simulink model "B1_IEEE_13_bus"  (R2022b)
settings: Solver=ode4  StartTime=0.0  StopTime=tend  FixedStep=ts  MaxStep=0.04  RelTol=1e-3
undefined symbols (not defined in the file): C, C_601, C_602, C_603, C_604, C_605, C_606, C_607, C_bc_ESS, C_bc_PV, C_bc_SC, C_SC_set, Cf, f0, fc, fc1, ft2km, fv, Gf, Idcbase, Ilim, J, Ki_c1, Ki_v, Kp_c1, Kp_v, L_601, L_602, L_603, L_604, L_605, L_606, L_607, L_bc_ESS, L_bc_PV, L_bc_SC, L_line_ESS, L_line_PV, Lf, Pnom, Pset_ESS, Pset_inv, Pset_load, Pset_PV, Pset_SC, Qset_inv, R_601, R_602, R_603, R_604, R_605, R_606, R_607, R_bc_ESS, R_bc_PV, R_bc_SC, R_line_ESS, R_line_PV, R_line_SC, Rf ... (+23)
libraries: spsSeriesRLCBranchLib x12, spsLoadFlowBusLib x12, spsPiSectionLineLib x9, spsThreePhaseSeriesRLCLoadLib x8, spsThreePhaseVIMeasurementLib x8, spsVoltageMeasurementLib x8, cstblocks x8, spsCurrentMeasurementLib x6, spsGroundLib x6, spsMultimeterLib x6, spsPowerLib x6, spsSeriesRLCLoadLib x5
(part 1 of 2)
settings Model: Creator=The MathWorks, Inc.  LastModifiedBy=hxq19
settings SolverCC: AlgebraicLoopSolver=TrustRegion
settings DataIOCC: ExternalInput=getinputstruct(op_IEEE_13_node_5)  InitialState=getstatestruct(op_IEEE_13_node_5)  LimitDataPoints=on  SaveFormat=Array  ReturnWorkspaceOutputs=off
settings OptimizationCC: LifeSpan=inf
settings DebuggingCC: AlgebraicLoopMsg=none  FcnCallInpInsideContextMsg=warning  StateNameClashWarn=warning  SFUnexpectedBacktrackingDiag=warning  SFNoUnconditionalDefaultTransitionDiag=warning  SFExecutionAtInitializationDiag=none  SFMachineParentedDataDiag=warning
settings ModelReferenceCC: EnableRefExpFcnMdlSchedulingChecks=on  PropagateSignalLabelsOutOfModel=off
settings SFSimCC: CustomCodeUndefinedFunction=UseInterfaceOnly
settings CodeAppCC: StateflowObjectComments=on
settings SimscapeCC: SimscapeNormalizeSystem=off

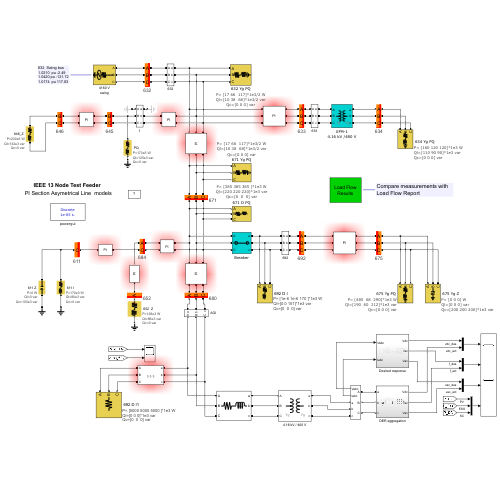
[thumbnail: Simulink's stored preview of the top-level diagram]
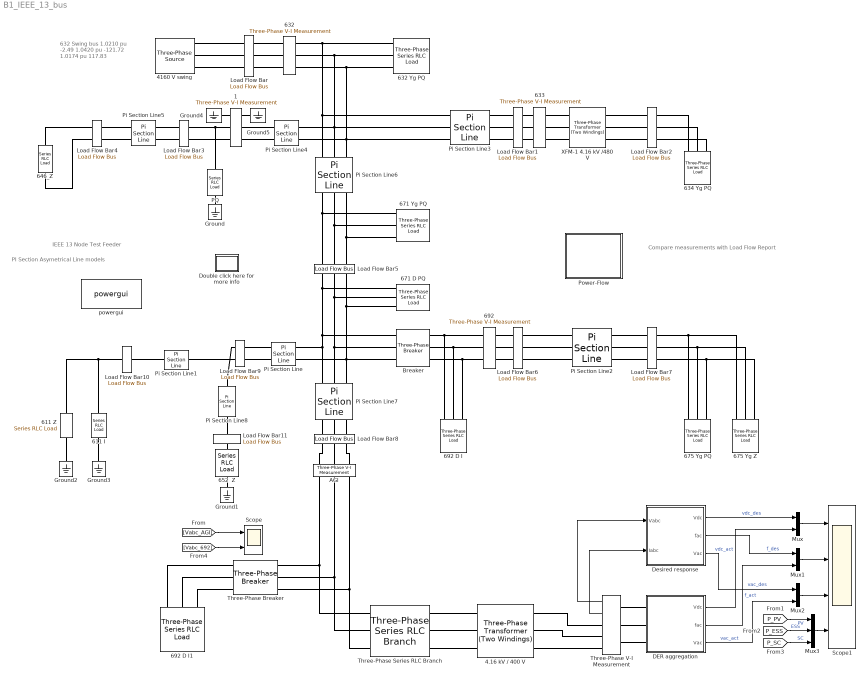
== system B1_IEEE_13_bus ==
  note: Compare measurements with
      | Load Flow Report
  note: 632 Swing bus
      | 1.0210 pu -2.49
      | 1.0420 pu -121.72
      | 1.0174 pu 117.83
  note: PI Section Asymetrical Line models
  note: IEEE 13 Node Test Feeder
  " 634 Yg PQ " : spsThreePhaseSeriesRLCLoadLib/Three-Phase Series RLC Load  LConnTagsString=A|B|C  Configuration=Y (grounded)  NominalVoltage=120e3  Vabc=[ 0.993926 1.02168 0.995885]*277.128  Vabcp=[1e3 1e3 1e3]  NominalFrequency=60  UnbalancedPower=on  ActivePower=1e+006  InductivePower=0  CapacitivePower=0  Pabc=[160 120 120]*1e3  QLabc=[110 90 90]*1e3  QCabc=[0 0 0]  Pabcp=[10e3 9e3 11e3]  QLabcp=[100 90 110]  QCabcp=[100 90 110]  Measurements=None  LoadType=constant PQ
      settings: AttributesFormatString=|
      | P= %<Pabc> W
      | Ql=%<QLabc> var
      | Qc=%<QCabc> var
  1 : spsThreePhaseVIMeasurementLib/Three-Phase V-I Measurement  VoltageMeasurement=phase-to-ground  SetLabelV=on  LabelV=Vabc_645  Vpu=off  VpuLL=off  CurrentMeasurement=yes  SetLabelI=on  LabelI=Iabc_645  Ipu=off  Pbase=100e6  Vbase=4160  OutputType=Complex  PhasorSimulation=off  PSBequivalent=0
  4.16 kV / 400 V : spsThreePhaseTransformerTwoWindingsLib/Three-Phase Transformer (Two Windings)  Winding1Connection=Yg  Winding2Connection=Yg  CoreType=Three single-phase transformers  SetSaturation=off  Hysteresis=off  DataFile='hysteresis'  SetInitialFlux=off  Measurements=None  UNITS=pu  NominalPower=[Stotal,f0]  Winding1=[ V1 , 0.001 , 0.03 ]  Winding2=[ V2 , 0.001 , 0.03 ]  Rm=500  Lm=inf  L0=0.5  Saturation=[ 0,0 ; 0.0024,1.2 ; 1.0,1.52 ]  InitialFluxes=[ 0.8 , -0.8 , 0.7 ]  BreakLoop=off  DiscreteSolver=Trapezoidal iterative  DataType=off  TransfoNumber=0
  4160 V swing : spsThreePhaseSourceLib/Three-Phase Source  InternalConnection=Yg  VoltagePhases=on  Voltage=120e3  PhaseAngle=0  Voltage_phases=[ 1.021 1.042 1.0174]*2401.78  PhaseAngles_phases=[ -2.49006 -121.72 117.83]  Frequency=60  NonIdealSource=on  SpecifyImpedance=off  Resistance=1e-5  Inductance=0  ShortCircuitLevel=100e6  BaseVoltage=120e3  XRratio=10  BusType=swing  Pref=0  Qref=0  Prefabc=[0 0 0]  Qrefabc=[0 0 0]  Qmin="[-inf  -inf -inf]"  Qmax="[inf  inf inf]"
  611 I : spsSeriesRLCLoadLib/Series RLC Load  LConnTagsString=a  RConnTagsString=__new0  NominalVoltage=0.986755*2401.78  NominalFrequency=60  ActivePower=170e3  InductivePower=80e3  CapacitivePower=0  Setx0=off  InitialVoltage=0  SetiL0=off  InitialCurrent=0  Measurements=Branch voltage and current  LoadType=constant I
      settings: AttributesFormatString=|
      | P=%<ActivePower> W
      | Ql=%<InductivePower> var
      | Qc=%<CapacitivePower> var
  611 Z : spsSeriesRLCLoadLib/Series RLC Load  LConnTagsString=a  RConnTagsString=__new0  NominalVoltage=4160/sqrt(3)  NominalFrequency=60  ActivePower=0  InductivePower=0  CapacitivePower=100e3  Setx0=off  InitialVoltage=0  SetiL0=off  InitialCurrent=0  Measurements=None  LoadType=constant Z
      settings: AttributesFormatString=|
      | P=%<ActivePower> W
      | Ql=%<InductivePower> var
      | Qc=%<CapacitivePower> var
  632 : spsThreePhaseVIMeasurementLib/Three-Phase V-I Measurement  VoltageMeasurement=phase-to-ground  SetLabelV=on  LabelV=Vabc_632  Vpu=off  VpuLL=off  CurrentMeasurement=yes  SetLabelI=on  LabelI=Iabc_632  Ipu=off  Pbase=100e6  Vbase=4160  OutputType=Complex  PhasorSimulation=off  PSBequivalent=0
  632 Yg PQ : spsThreePhaseSeriesRLCLoadLib/Three-Phase Series RLC Load  LConnTagsString=A|B|C  Configuration=Y (grounded)  NominalVoltage=120e3  Vabc=[ 1.021 1.042 1.0174]*2401.78  Vabcp=[1e3 1e3 1e3]  NominalFrequency=60  UnbalancedPower=on  ActivePower=1e+006  InductivePower=0  CapacitivePower=0  Pabc="[17 66  117]*1e3/2"  QLabc="[10 38  68]*1e3/2"  QCabc=[0 0 0]  Pabcp=[10e3 9e3 11e3]  QLabcp=[100 90 110]  QCabcp=[100 90 110]  Measurements=None  LoadType=constant PQ
      settings: AttributesFormatString=|
      | P= %<Pabc> W
      | Ql=%<QLabc> var
      | Qc=%<QCabc> var
  633 : spsThreePhaseVIMeasurementLib/Three-Phase V-I Measurement  VoltageMeasurement=phase-to-ground  SetLabelV=on  LabelV=Vabc_633  Vpu=off  VpuLL=off  CurrentMeasurement=yes  SetLabelI=on  LabelI=Iabc_633  Ipu=off  Pbase=100e6  Vbase=4160  OutputType=Complex  PhasorSimulation=off  PSBequivalent=0
  646_Z : spsSeriesRLCLoadLib/Series RLC Load  LConnTagsString=a  RConnTagsString=__new0  NominalVoltage=4160  NominalFrequency=60  ActivePower=230e3  InductivePower=132e3  CapacitivePower=0  Setx0=off  InitialVoltage=0  SetiL0=off  InitialCurrent=0  Measurements=None  LoadType=constant Z
      settings: AttributesFormatString=|
      | P=%<ActivePower> W
      | Ql=%<InductivePower> var
      | Qc=%<CapacitivePower> var
  "652  Z " : spsSeriesRLCLoadLib/Series RLC Load  LConnTagsString=a  RConnTagsString=__new0  NominalVoltage=4160/sqrt(3)  NominalFrequency=60  ActivePower=128e3  InductivePower=86e3  CapacitivePower=0  Setx0=off  InitialVoltage=0  SetiL0=off  InitialCurrent=0  Measurements=None  LoadType=constant Z
      settings: AttributesFormatString=|
      | P=%<ActivePower> W
      | Ql=%<InductivePower> var
      | Qc=%<CapacitivePower> var
  671 D PQ : spsThreePhaseSeriesRLCLoadLib/Three-Phase Series RLC Load  LConnTagsString=A|B|C  Configuration=Delta  NominalVoltage=120e3  Vabc="[1  1  1]*120e3/sqrt(3)"  Vabcp=[ 1.7426 1.77325 1.71534]*2401.78  NominalFrequency=60  UnbalancedPower=on  ActivePower=1e+006  InductivePower=0  CapacitivePower=0  Pabc="[17 66  117]*1e3/2"  QLabc="[10 38  68]*1e3/2"  QCabc=[0 0 0]  Pabcp=[385 385 385 ]*1e3  QLabcp=[220 220 220]*1e3  QCabcp="[0  0  0]"  Measurements=Branch voltages and currents  LoadType=constant PQ
      settings: AttributesFormatString=|
      | P= %<Pabcp> W
      | Ql=%<QLabcp> var
      | Qc=%<QCabcp> var
  671 Yg PQ : spsThreePhaseSeriesRLCLoadLib/Three-Phase Series RLC Load  LConnTagsString=A|B|C  Configuration=Y (grounded)  NominalVoltage=120e3  Vabc=[ 0.990007 1.05293 0.977696]*2401.78  Vabcp=[1e3 1e3 1e3]  NominalFrequency=60  UnbalancedPower=on  ActivePower=1e+006  InductivePower=0  CapacitivePower=0  Pabc="[17 66  117]*1e3/2"  QLabc="[10 38  68]*1e3/2"  QCabc=[0 0 0]  Pabcp=[10e3 9e3 11e3]  QLabcp=[100 90 110]  QCabcp=[100 90 110]  Measurements=None  LoadType=constant PQ
      settings: AttributesFormatString=|
      | P= %<Pabc> W
      | Ql=%<QLabc> var
      | Qc=%<QCabc> var
  675 Yg PQ : spsThreePhaseSeriesRLCLoadLib/Three-Phase Series RLC Load  LConnTagsString=A|B|C  Configuration=Y (grounded)  NominalVoltage=120e3  Vabc=[ 0.983621 1.05532 0.975578]*2401.78  Vabcp=[1e3 1e3 1e3]  NominalFrequency=60  UnbalancedPower=on  ActivePower=1e+006  InductivePower=0  CapacitivePower=0  Pabc="[485  68  290]*1e3"  QLabc="[190  60  212]*1e3"  QCabc=[0 0 0]  Pabcp=[10e3 9e3 11e3]  QLabcp=[100 90 110]  QCabcp=[100 90 110]  Measurements=Branch voltages and currents  LoadType=constant PQ
      settings: AttributesFormatString=|
      | P= %<Pabc> W
      | Ql=%<QLabc> var
      | Qc=%<QCabc> var
  675 Yg Z : spsThreePhaseSeriesRLCLoadLib/Three-Phase Series RLC Load  LConnTagsString=A|B|C  Configuration=Y (grounded)  NominalVoltage=120e3  Vabc="[1  1  1]*4160/sqrt(3)"  Vabcp=[1e3 1e3 1e3]  NominalFrequency=60  UnbalancedPower=on  ActivePower=1e+006  InductivePower=0  CapacitivePower=0  Pabc=[0 0 0]  QLabc=[0 0 0]  QCabc=[200 200 200]*1e3  Pabcp=[10e3 9e3 11e3]  QLabcp=[100 90 110]  QCabcp=[100 90 110]  Measurements=None  LoadType=constant Z
      settings: AttributesFormatString=|
      | P= %<Pabc> W
      | Ql=%<QLabc> var
      | Qc=%<QCabc> var
  692 : spsThreePhaseVIMeasurementLib/Three-Phase V-I Measurement  VoltageMeasurement=phase-to-ground  SetLabelV=on  LabelV=Vabc_692  Vpu=off  VpuLL=off  CurrentMeasurement=yes  SetLabelI=on  LabelI=Iabc_692  Ipu=off  Pbase=100e6  Vbase=4160  OutputType=Complex  PhasorSimulation=off  PSBequivalent=0
  692 D I : spsThreePhaseSeriesRLCLoadLib/Three-Phase Series RLC Load  LConnTagsString=A|B|C  Configuration=Delta  NominalVoltage=120e3  Vabc="[1  1  1]*120e3/sqrt(3)"  Vabcp=[ 1.73731 1.75253 1.72367]*2401.78  NominalFrequency=60  UnbalancedPower=on  ActivePower=1e+006  InductivePower=0  CapacitivePower=0  Pabc="[17 66  117]*1e3/2"  QLabc="[10 38  68]*1e3/2"  QCabc=[0 0 0]  Pabcp=[1e-6 1e-6 170 ]*1e3  QLabcp=[0 0 151]*1e3  QCabcp="[0  0  0]"  Measurements=Branch voltages and currents  LoadType=constant I
      settings: AttributesFormatString=|
      | P= %<Pabcp> W
      | Ql=%<QLabcp> var
      | Qc=%<QCabcp> var
  692 D I1 : spsThreePhaseSeriesRLCLoadLib/Three-Phase Series RLC Load  LConnTagsString=A|B|C  Configuration=Delta  NominalVoltage=120e3  Vabc="[1  1  1]*120e3/sqrt(3)"  Vabcp=[ 1.73731 1.75253 1.72367]*2401.78  NominalFrequency=60  UnbalancedPower=on  ActivePower=1e+006  InductivePower=0  CapacitivePower=0  Pabc="[17 66  117]*1e3/2"  QLabc="[10 38  68]*1e3/2"  QCabc=[0 0 0]  Pabcp=[5000 5000 5000 ]*1e3  QLabcp=[0 0 0]*1e3  QCabcp="[0  0  0]"  Measurements=Branch voltages and currents  LoadType=constant I
      settings: AttributesFormatString=|
      | P= %<Pabcp> W
      | Ql=%<QLabcp> var
      | Qc=%<QCabcp> var
  AGI : spsThreePhaseVIMeasurementLib/Three-Phase V-I Measurement  VoltageMeasurement=phase-to-ground  SetLabelV=on  LabelV=Vabc_AGI  Vpu=off  VpuLL=off  CurrentMeasurement=yes  SetLabelI=on  LabelI=Iabc_AGI  Ipu=off  Pbase=100e6  Vbase=4160  OutputType=Complex  PhasorSimulation=off  PSBequivalent=0
  Breaker : spsThreePhaseBreakerLib/Three-Phase Breaker  InitialState=closed  SwitchA=off  SwitchB=off  SwitchC=off  SwitchTimes=[0.5 ]  External=off  BreakerResistance=0.0001  SnubberResistance=inf  SnubberCapacitance=0  Measurements=None
  DER aggregation : Subsystem
      settings: PortSchema="{\"entries\":[{\"content\":{\"sides\":[{\"content\":{\"connectorIds\":[\"Out1\",\"Out2\",\"Out3\"]},\"type\":\"ConnectorPlacement.EquallySpacedRectSide\",\"uuid\":\"d17645c7-cdec-4633-b3c6-cd15445995c3\"},{\"content\":{\"connectorIds\":[\"RConn1\",\"RConn2\",\"RConn3\"],\"side\":\"RIGHT\"},\"type\":\"ConnectorPlacement.EquallySpacedRectSide\",\"uuid\":\"25a3cf30-901e-4740-a075-3c8408526c60\"},{\"content\":{\"connectorIds\":[],\"side\":\"TOP\"},\"type\":\"ConnectorPlacement.EquallySpacedRectSide\",\"uuid\":\"8cde02ff-980e-4e20-bc67-22f4d69f4d72\"}]},\"type\":\"ConnectorPlacement.EquallySpacedConnector\",\"uuid\":\"2536287c-4269-40cd-b41b-6d4dfba348bd\"}],\"packageUris\":[\"http://schema.mathworks.com/mf0/Connector/R2020b\"],\"version\":\"1.0\"}"
  Desired response : Subsystem
      settings: PortSchema="{\"entries\":[{\"content\":{\"sides\":[{\"content\":{\"connectorIds\":[\"Out1\",\"Out2\",\"Out3\"]},\"type\":\"ConnectorPlacement.EquallySpacedRectSide\",\"uuid\":\"d17645c7-cdec-4633-b3c6-cd15445995c3\"},{\"content\":{\"connectorIds\":[\"In1\",\"In2\"],\"side\":\"RIGHT\"},\"type\":\"ConnectorPlacement.EquallySpacedRectSide\",\"uuid\":\"25a3cf30-901e-4740-a075-3c8408526c60\"},{\"content\":{\"connectorIds\":[],\"side\":\"TOP\"},\"type\":\"ConnectorPlacement.EquallySpacedRectSide\",\"uuid\":\"8cde02ff-980e-4e20-bc67-22f4d69f4d72\"}]},\"type\":\"ConnectorPlacement.EquallySpacedConnector\",\"uuid\":\"2536287c-4269-40cd-b41b-6d4dfba348bd\"}],\"packageUris\":[\"http://schema.mathworks.com/mf0/Connector/R2020b\"],\"version\":\"1.0\"}"
  Double click here for more info : Subsystem
      settings: OpenFcn=showdemo(bdroot(gcb))
      mask Display: disp('?')
  Ground{,1..5} (6 alike) : spsGroundLib/Ground  LConnTagsString=a
  Load Flow Bar : spsLoadFlowBusLib/Load Flow Bus  LConnTagsString=a|b|c  RConnTagsString=a|b|c  Phases=ABC  Connectors=on both sides  ID=632  Vbase=4160/sqrt(3)  Vref="[ 1.0210  1.0420  1.0174]"  Vangle="[ -2.49  -121.72  117.83]"  VLF=1.021  VLFb=1.042  VLFc=1.017  angleLF=-2.49  angleLFb=-121.7  angleLFc=117.8
      settings: AttributesFormatString=%<ID>
  Load Flow Bar1 : spsLoadFlowBusLib/Load Flow Bus  LConnTagsString=a|b|c  RConnTagsString=a|b|c  Phases=ABC  Connectors=on both sides  ID=633  Vbase=4160/sqrt(3)  Vref=[1.0 1.0 1.0]  Vangle=[0 -120 120]  VLF=1.018  VLFb=1.04  VLFc=1.015  angleLF=-2.555  angleLFb=-121.8  angleLFc=117.8
      settings: AttributesFormatString=%<ID>
  Load Flow Bar10 : spsLoadFlowBusLib/Load Flow Bus  LConnTagsString=a  RConnTagsString=a  Phases=C  Connectors=on both sides  ID=611  Vbase=4160/sqrt(3)  Vref=1.0  Vangle=0  VLF=NaN  VLFb=NaN  VLFc=0.9737  angleLF=NaN  angleLFb=NaN  angleLFc=115.8
      settings: AttributesFormatString=%<ID>
  Load Flow Bar11 : spsLoadFlowBusLib/Load Flow Bus  LConnTagsString=a  RConnTagsString=a  Phases=A  Connectors=on both sides  ID=652  Vbase=4160/sqrt(3)  Vref=1.0  Vangle=0  VLF=0.9825  VLFb=NaN  VLFc=NaN  angleLF=-5.246  angleLFb=NaN  angleLFc=NaN
      settings: AttributesFormatString=%<ID>
  Load Flow Bar2 : spsLoadFlowBusLib/Load Flow Bus  LConnTagsString=a|b|c  RConnTagsString=a|b|c  Phases=ABC  Connectors=on both sides  ID=634  Vbase=480/sqrt(3)  Vref=[1.0 1.0 1.0]  Vangle=[0 -120 120]  VLF=0.9939  VLFb=1.022  VLFc=0.9959  angleLF=-3.232  angleLFb=-122.2  angleLFc=117.3
      settings: AttributesFormatString=%<ID>
  Load Flow Bar3 : spsLoadFlowBusLib/Load Flow Bus  LConnTagsString=a|b  RConnTagsString=a|b  Phases=BC  Connectors=on both sides  ID=645  Vbase=4160/sqrt(3)  Vref=[1.0 1.0 ]  Vangle=[0 0]  VLF=NaN  VLFb=1.033  VLFc=1.015  angleLF=NaN  angleLFb=-121.9  angleLFc=117.9
      settings: AttributesFormatString=%<ID>
  Load Flow Bar4 : spsLoadFlowBusLib/Load Flow Bus  LConnTagsString=a|b  RConnTagsString=a|b  Phases=BC  Connectors=on both sides  ID=646  Vbase=4160/sqrt(3)  Vref=[1.0 1.0 ]  Vangle=[0 0]  VLF=NaN  VLFb=1.031  VLFc=1.013  angleLF=NaN  angleLFb=-122  angleLFc=117.9
      settings: AttributesFormatString=%<ID>
  Load Flow Bar5 : spsLoadFlowBusLib/Load Flow Bus  LConnTagsString=a|b|c  RConnTagsString=a|b|c  Phases=ABC  Connectors=on both sides  ID=671  Vbase=4160/sqrt(3)  Vref=[1.0 1.0 1.0]  Vangle=[0 -120 120]  VLF=0.99  VLFb=1.053  VLFc=0.9777  angleLF=-5.298  angleLFb=-122.3  angleLFc=116
      settings: AttributesFormatString=%<ID>
  Load Flow Bar6 : spsLoadFlowBusLib/Load Flow Bus  LConnTagsString=a|b|c  RConnTagsString=a|b|c  Phases=ABC  Connectors=on both sides  ID=692  Vbase=4160/sqrt(3)  Vref=[1.0 1.0 1.0]  Vangle=[0 -120 120]  VLF=0.99  VLFb=1.053  VLFc=0.9777  angleLF=-5.298  angleLFb=-122.3  angleLFc=116
      settings: AttributesFormatString=%<ID>
  Load Flow Bar7 : spsLoadFlowBusLib/Load Flow Bus  LConnTagsString=a|b|c  RConnTagsString=a|b|c  Phases=ABC  Connectors=on both sides  ID=675  Vbase=4160/sqrt(3)  Vref=[1.0 1.0 1.0]  Vangle=[0 -120 120]  VLF=0.9836  VLFb=1.055  VLFc=0.9756  angleLF=-5.544  angleLFb=-122.5  angleLFc=116
      settings: AttributesFormatString=%<ID>
  Load Flow Bar8 : spsLoadFlowBusLib/Load Flow Bus  LConnTagsString=a|b|c  RConnTagsString=a|b|c  Phases=ABC  Connectors=on both sides  ID=680  Vbase=4160/sqrt(3)  Vref=[1.0 1.0 1.0]  Vangle=[0 -120 120]  VLF=0.99  VLFb=1.053  VLFc=0.9777  angleLF=-5.298  angleLFb=-122.3  angleLFc=116
      settings: AttributesFormatString=%<ID>
  Load Flow Bar9 : spsLoadFlowBusLib/Load Flow Bus  LConnTagsString=a|b  RConnTagsString=a|b  Phases=AC  Connectors=on both sides  ID=684  Vbase=4160/sqrt(3)  Vref=[1.0 1.0 ]  Vangle=[0 -120 ]  VLF=0.9881  VLFb=NaN  VLFc=0.9757  angleLF=-5.321  angleLFb=NaN  angleLFc=115.9
      settings: AttributesFormatString=%<ID>
  Mux : Mux  Inputs=2
  Mux1 : Mux  Inputs=2
  Mux2 : Mux  Inputs=2
  Mux3 : Mux  Inputs=3
  PQ : spsSeriesRLCLoadLib/Series RLC Load  LConnTagsString=a  RConnTagsString=__new0  NominalVoltage=1.03283*2401.78  NominalFrequency=60  ActivePower=170e3  InductivePower=125e3  CapacitivePower=0  Setx0=off  InitialVoltage=0  SetiL0=off  InitialCurrent=0  Measurements=None  LoadType=constant PQ
      settings: AttributesFormatString=|
      | P=%<ActivePower> W
      | Ql=%<InductivePower> var
      | Qc=%<CapacitivePower> var
  Pi Section Line : spsPiSectionLineLib/Pi Section Line  LConnTagsString=1|i2  RConnTagsString=1|o2  Phases=2  PiSections=1  Length=300*ft2km  Frequency=60  Resistance=R_604([1 3],[1 3])  Inductance=L_604([1 3],[1 3])  Capacitance=C_604([1 3],[1 3])  SpecifyConductance=off  Conductance=0  Measurements=None  Measurements2=None
      settings: LibrarySourceBlock=sps_lib/Power Grid Elements/Pi Section Line
  Pi Section Line1 : spsPiSectionLineLib/Pi Section Line  LConnTagsString=1  RConnTagsString=1  Phases=1  PiSections=1  Length=300*ft2km  Frequency=60  Resistance=R_605(3,3)  Inductance=L_605(3,3)  Capacitance=C_605(3,3)  SpecifyConductance=off  Conductance=0  Measurements=None  Measurements2=None
      settings: LibrarySourceBlock=sps_lib/Power Grid Elements/Pi Section Line
  Pi Section Line2 : spsPiSectionLineLib/Pi Section Line  LConnTagsString=1|i2|i3  RConnTagsString=1|o2|o3  Phases=3  PiSections=1  Length=500*ft2km  Frequency=60  Resistance=R_606  Inductance=L_606  Capacitance=C_606  SpecifyConductance=off  Conductance=0  Measurements=None  Measurements2=None
      settings: LibrarySourceBlock=sps_lib/Power Grid Elements/Pi Section Line
  Pi Section Line3 : spsPiSectionLineLib/Pi Section Line  LConnTagsString=1|i2|i3  RConnTagsString=1|o2|o3  Phases=3  PiSections=1  Length=500*ft2km  Frequency=60  Resistance=R_602  Inductance=L_602  Capacitance=C_602  SpecifyConductance=off  Conductance=0  Measurements=None  Measurements2=None
      settings: LibrarySourceBlock=sps_lib/Power Grid Elements/Pi Section Line
  Pi Section Line4 : spsPiSectionLineLib/Pi Section Line  LConnTagsString=1|i2  RConnTagsString=1|o2  Phases=2  PiSections=1  Length=500*ft2km  Frequency=60  Resistance=R_603(2:3,2:3)  Inductance=L_603(2:3,2:3)  Capacitance=C_603(2:3,2:3)  SpecifyConductance=off  Conductance=0  Measurements=None  Measurements2=None
      settings: LibrarySourceBlock=sps_lib/Power Grid Elements/Pi Section Line
  Pi Section Line5 : spsPiSectionLineLib/Pi Section Line  LConnTagsString=1|i2  RConnTagsString=1|o2  Phases=2  PiSections=1  Length=300*ft2km  Frequency=60  Resistance=R_603(2:3,2:3)  Inductance=L_603(2:3,2:3)  Capacitance=C_603(2:3,2:3)  SpecifyConductance=off  Conductance=0  Measurements=None  Measurements2=None
      settings: LibrarySourceBlock=sps_lib/Power Grid Elements/Pi Section Line
  Pi Section Line6 : spsPiSectionLineLib/Pi Section Line  LConnTagsString=1|i2|i3  RConnTagsString=1|o2|o3  Phases=3  PiSections=1  Length=2000*ft2km  Frequency=60  Resistance=R_601  Inductance=L_601  Capacitance=C_601  SpecifyConductance=off  Conductance=0  Measurements=None  Measurements2=None
      settings: LibrarySourceBlock=sps_lib/Power Grid Elements/Pi Section Line
  Pi Section Line7 : spsPiSectionLineLib/Pi Section Line  LConnTagsString=1|i2|i3  RConnTagsString=1|o2|o3  Phases=3  PiSections=1  Length=1000*ft2km  Frequency=60  Resistance=R_601  Inductance=L_601  Capacitance=C_601  SpecifyConductance=off  Conductance=0  Measurements=None  Measurements2=None
      settings: LibrarySourceBlock=sps_lib/Power Grid Elements/Pi Section Line
  Pi Section Line8 : spsPiSectionLineLib/Pi Section Line  LConnTagsString=1  RConnTagsString=1  Phases=1  PiSections=1  Length=800*ft2km  Frequency=60  Resistance=R_607(1,1)  Inductance=L_607(1,1)  Capacitance=C_607(1,1)  SpecifyConductance=off  Conductance=0  Measurements=None  Measurements2=None
      settings: LibrarySourceBlock=sps_lib/Power Grid Elements/Pi Section Line
  Power-Flow : Subsystem
      mask Display: disp('Load Flow\nResults')
  Scope : Scope  NumInputPorts=2
  Scope1 : Scope  NumInputPorts=4
  Three-Phase Series RLC Branch : spsThreePhaseSeriesRLCBranchLib/Three-Phase Series RLC Branch  LConnTagsString=A|B|C  RConnTagsString=A|B|C  BranchType=RL  Resistance=Rg*Zbase  Inductance=Zg*Zbase/w0  Capacitance=1e-6  Measurements=None
  Three-Phase V-I Measurement : spsThreePhaseVIMeasurementLib/Three-Phase V-I Measurement  VoltageMeasurement=phase-to-ground  SetLabelV=off  LabelV=Vabc  Vpu=off  VpuLL=off  CurrentMeasurement=yes  SetLabelI=off  LabelI=Iabc  Ipu=off  Pbase=Sbase  Vbase=V2  OutputType=Complex  PhasorSimulation=off  PSBequivalent=0
  Three-Phase Breaker : spsThreePhaseBreakerLib/Three-Phase Breaker  InitialState=open  SwitchA=on  SwitchB=on  SwitchC=on  SwitchTimes="[tdist  trcv]"  External=off  BreakerResistance=0.01  SnubberResistance=1e6  SnubberCapacitance=inf  Measurements=None
  XFM-1 4.16 kV /480 V : spsThreePhaseTransformerTwoWindingsLib/Three-Phase Transformer (Two Windings)  Winding1Connection=Yg  Winding2Connection=Yg  CoreType=Three single-phase transformers  SetSaturation=off  Hysteresis=off  DataFile='hysteresis'  SetInitialFlux=off  Measurements=None  UNITS=pu  NominalPower=[ 500e3 , 60 ]  Winding1=[4160 0.011 0.02]  Winding2=[480 0 0]  Rm=500  Lm=500  L0=0.5  Saturation=[0 0;0.0024 1.2;1 1.52]  InitialFluxes=[0.8 -0.8 0.7]  BreakLoop=off  DiscreteSolver=Trapezoidal iterative  DataType=off  TransfoNumber=1
  powergui : spspowerguiLib/powergui  Priority=1  SimulationMode=Discrete  SampleTime=1e-5  frequency=60  Iterations=50  frequencyindice=60  Pbase=100e3  ErrMax=0.0001  UnitsV=kV  UnitsW=kW  buscounter=0  FunctionMessages=off  echomessages=off  EnableUseOfTLC=off  CurrentSourceSwitches=off  DisableSnubberDevices=off  DisableRonSwitches=off  DisableVfSwitches=off  DisplayEquations=off  AutomaticDiscreteSolvers=off  SolverType=Tustin/Backward Euler (TBE)  Interpol=off  ExternalGateDelay=off  methode=off  Ts=0  x0status=blocks  SPID=off  SwTol=0  HookPort=off  NonlinearTolerance=1e-4  nMaxIteration=100  ContinueOnMaxIteration=off  RestoreLinks=warning  ResistiveCurrentMeasurement=off  Frange=[0:2:500]  Ylog=off  Xlog=on  ShowGrid=off  save=off  variable=ZData  structure=0  ZoomFFT=on  StartTime=0.0  cycles=1  DisplayStyle=1  fundamental=60  FreqAxis=off  MaxFrequency=1000  frequencyindicesteady=1  RmsSteady=1  display=off
  wires:
  [Vabc_AGI] -> Scope/1
  [P_SC] -> Mux3/3  "SC"
  DER aggregation/1(Vdc) -> Mux/2  "vdc_act"
  DER aggregation/2(fac) -> Mux1/2  "f_act"
  Mux3/1 -> Scope1/4
  Three-Phase V-I Measurement/1 -> Desired response/1(Vabc)
  [P_PV] -> Mux3/1  "PV"
  [P_ESS] -> Mux3/2  "ESS"
  DER aggregation/3(Vac) -> Mux2/2  "vac_act"
  Mux/1 -> Scope1/1
  Mux1/1 -> Scope1/2
  Desired response/2(fac) -> Mux1/1  "f_des"
  Desired response/3(Vac) -> Mux2/1  "vac_des"
  Desired response/1(Vdc) -> Mux/1  "vdc_des"
  Mux2/1 -> Scope1/3
  Three-Phase V-I Measurement/2 -> Desired response/2(Iabc)
  [Vabc_692] -> Scope/2
  connections:
  632/RConn2 -- 632 Yg PQ/LConn2 -- Pi Section Line4/RConn1 -- Pi Section Line6/LConn2 -- Pi Section Line3/LConn2
  675 Yg Z/LConn1 -- Load Flow Bar7/LConn1 -- 675 Yg PQ/LConn1
  671 D PQ/LConn2 -- Breaker/LConn2 -- Pi Section Line7/LConn2 -- Load Flow Bar5/RConn2
  Breaker/RConn3 -- 692 D I/LConn3 -- 692/LConn3
  Pi Section Line/RConn1 -- Pi Section Line7/LConn1 -- 671 D PQ/LConn1 -- Load Flow Bar5/RConn1 -- Breaker/LConn1
  Load Flow Bar3/RConn1 -- 1/LConn2 -- PQ/LConn1
  675 Yg Z/LConn3 -- Load Flow Bar7/LConn3 -- 675 Yg PQ/LConn3
  671 Yg PQ/LConn2 -- Load Flow Bar5/LConn2 -- Pi Section Line6/RConn2
  Load Flow Bar10/LConn1 -- 611 Z/LConn1 -- 611 I/LConn1
  671 Yg PQ/LConn3 -- Load Flow Bar5/LConn3 -- Pi Section Line6/RConn3
  Pi Section Line6/LConn1 -- 632 Yg PQ/LConn1 -- 632/RConn1 -- Pi Section Line3/LConn1
  671 D PQ/LConn3 -- Load Flow Bar5/RConn3 -- Pi Section Line7/LConn3 -- Breaker/LConn3 -- Pi Section Line/RConn2
  632/RConn3 -- 632 Yg PQ/LConn3 -- Pi Section Line4/RConn2 -- Pi Section Line6/LConn3 -- Pi Section Line3/LConn3
  Breaker/RConn1 -- 692 D I/LConn1 -- 692/LConn1
  671 Yg PQ/LConn1 -- Load Flow Bar5/LConn1 -- Pi Section Line6/RConn1
  Breaker/RConn2 -- 692 D I/LConn2 -- 692/LConn2
  675 Yg Z/LConn2 -- Load Flow Bar7/LConn2 -- 675 Yg PQ/LConn2
  692/RConn1 -- Load Flow Bar6/RConn1
  1/LConn3 -- Load Flow Bar3/RConn2
  Ground2/LConn1 -- 611 Z/RConn1
  Pi Section Line1/LConn1 -- Load Flow Bar10/RConn1
  692/RConn3 -- Load Flow Bar6/RConn3
  Pi Section Line5/RConn1 -- Load Flow Bar3/LConn1
  Load Flow Bar2/LConn2 -- XFM-1 4.16 kV /480 V/RConn2
  " 634 Yg PQ "/LConn2 -- Load Flow Bar2/RConn2
  4160 V swing/RConn2 -- Load Flow Bar/LConn2
  Pi Section Line2/RConn3 -- Load Flow Bar7/RConn3
  Pi Section Line7/RConn3 -- Load Flow Bar8/LConn3
  Pi Section Line5/RConn2 -- Load Flow Bar3/LConn2
  633/LConn1 -- Load Flow Bar1/RConn1
  Pi Section Line2/RConn1 -- Load Flow Bar7/RConn1
  Ground/LConn1 -- PQ/RConn1
  Pi Section Line/LConn1 -- Load Flow Bar9/RConn1
  Pi Section Line7/RConn1 -- Load Flow Bar8/LConn1
  Load Flow Bar4/LConn2 -- 646_Z/RConn1
  1/RConn3 -- Pi Section Line4/LConn2
  Pi Section Line5/LConn1 -- Load Flow Bar4/RConn1
  Pi Section Line7/RConn2 -- Load Flow Bar8/LConn2
  Pi Section Line8/LConn1 -- Load Flow Bar9/LConn1
  692/RConn2 -- Load Flow Bar6/RConn2
  Ground1/LConn1 -- "652  Z "/RConn1
  Pi Section Line2/LConn1 -- Load Flow Bar6/LConn1
  4160 V swing/RConn1 -- Load Flow Bar/LConn1
  Pi Section Line/LConn2 -- Load Flow Bar9/RConn2
  633/RConn3 -- XFM-1 4.16 kV /480 V/LConn3
  Pi Section Line8/RConn1 -- Load Flow Bar11/LConn1
  4160 V swing/RConn3 -- Load Flow Bar/LConn3
  "652  Z "/LConn1 -- Load Flow Bar11/RConn1
  633/RConn2 -- XFM-1 4.16 kV /480 V/LConn2
  1/RConn1 -- Ground5/LConn1
  633/RConn1 -- XFM-1 4.16 kV /480 V/LConn1
  Pi Section Line2/LConn2 -- Load Flow Bar6/LConn2
  Load Flow Bar/RConn2 -- 632/LConn2
  Ground3/LConn1 -- 611 I/RConn1
  Pi Section Line3/RConn1 -- Load Flow Bar1/LConn1
  Load Flow Bar/RConn1 -- 632/LConn1
  Pi Section Line5/LConn2 -- Load Flow Bar4/RConn2
  Pi Section Line2/RConn2 -- Load Flow Bar7/RConn2
  Pi Section Line3/RConn2 -- Load Flow Bar1/LConn2
  633/LConn3 -- Load Flow Bar1/RConn3
  Load Flow Bar/RConn3 -- 632/LConn3
  Pi Section Line3/RConn3 -- Load Flow Bar1/LConn3
  633/LConn2 -- Load Flow Bar1/RConn2
  Ground4/LConn1 -- 1/LConn1
  Pi Section Line1/RConn1 -- Load Flow Bar9/LConn2
  Load Flow Bar2/LConn1 -- XFM-1 4.16 kV /480 V/RConn1
  " 634 Yg PQ "/LConn1 -- Load Flow Bar2/RConn1
  Pi Section Line2/LConn3 -- Load Flow Bar6/LConn3
  Load Flow Bar2/LConn3 -- XFM-1 4.16 kV /480 V/RConn3
  1/RConn2 -- Pi Section Line4/LConn1
  " 634 Yg PQ "/LConn3 -- Load Flow Bar2/RConn3
  646_Z/LConn1 -- Load Flow Bar4/LConn1
  AGI/RConn1 -- Load Flow Bar8/RConn1
  AGI/RConn2 -- Load Flow Bar8/RConn2
  AGI/RConn3 -- Load Flow Bar8/RConn3
  4.16 kV / 400 V/RConn1 -- Three-Phase V-I Measurement/RConn1
  4.16 kV / 400 V/RConn3 -- Three-Phase V-I Measurement/RConn3
  DER aggregation/RConn1 -- Three-Phase V-I Measurement/LConn1
  Three-Phase V-I Measurement/RConn2 -- 4.16 kV / 400 V/RConn2
  DER aggregation/RConn2 -- Three-Phase V-I Measurement/LConn2
  DER aggregation/RConn3 -- Three-Phase V-I Measurement/LConn3
  Three-Phase Series RLC Branch/RConn1 -- 4.16 kV / 400 V/LConn1
  Three-Phase Series RLC Branch/RConn2 -- 4.16 kV / 400 V/LConn2
  Three-Phase Series RLC Branch/RConn3 -- 4.16 kV / 400 V/LConn3
  Three-Phase Series RLC Branch/LConn1 -- Three-Phase Breaker/RConn1 -- AGI/LConn1
  Three-Phase Series RLC Branch/LConn2 -- Three-Phase Breaker/RConn2 -- AGI/LConn2
  AGI/LConn3 -- Three-Phase Series RLC Branch/LConn3 -- Three-Phase Breaker/RConn3
  692 D I1/LConn1 -- Three-Phase Breaker/LConn1
  Three-Phase Breaker/LConn2 -- 692 D I1/LConn2
  692 D I1/LConn3 -- Three-Phase Breaker/LConn3

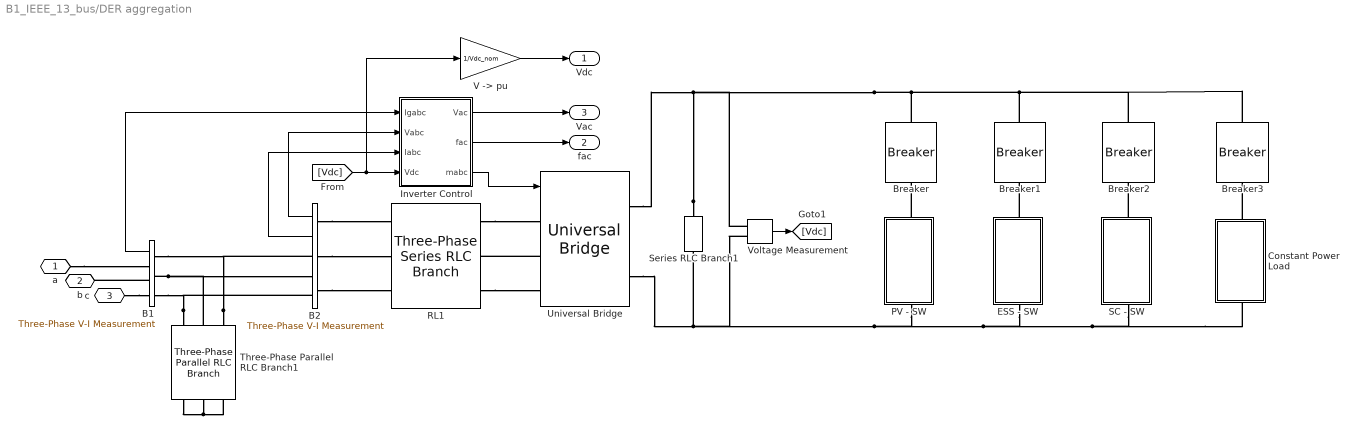
== system B1_IEEE_13_bus/DER aggregation ==
  B1 : spsThreePhaseVIMeasurementLib/Three-Phase V-I Measurement  VoltageMeasurement=no  SetLabelV=off  LabelV=Vabc_B1  Vpu=off  VpuLL=off  CurrentMeasurement=yes  SetLabelI=off  LabelI=Iabc_B1  Ipu=off  Pbase=100e6  Vbase=500e3  OutputType=Magnitude  PhasorSimulation=off  PSBequivalent=0
  B2 : spsThreePhaseVIMeasurementLib/Three-Phase V-I Measurement  VoltageMeasurement=phase-to-ground  SetLabelV=off  LabelV=Vabc_B1  Vpu=off  VpuLL=off  CurrentMeasurement=yes  SetLabelI=off  LabelI=Iabc_B1  Ipu=off  Pbase=100e6  Vbase=500e3  OutputType=Magnitude  PhasorSimulation=off  PSBequivalent=0
  Breaker : spsBreakerLib/Breaker  InitialState=0  SwitchingTimes=tPVconnect  External=off  BreakerResistance=1e-6  SnubberResistance=1e6  SnubberCapacitance=inf  Measurements=None  MoreParameters=on  NoBreakLoop=off
  Breaker1 : spsBreakerLib/Breaker  InitialState=0  SwitchingTimes=tESSconnect  External=off  BreakerResistance=1e-6  SnubberResistance=1e6  SnubberCapacitance=inf  Measurements=None  MoreParameters=on  NoBreakLoop=off
  Breaker2 : spsBreakerLib/Breaker  InitialState=0  SwitchingTimes=tSCconnect  External=off  BreakerResistance=1e-6  SnubberResistance=1e6  SnubberCapacitance=inf  Measurements=None  MoreParameters=on  NoBreakLoop=off
  Breaker3 : spsBreakerLib/Breaker  InitialState=0  SwitchingTimes=tLoadconnect  External=off  BreakerResistance=1e-6  SnubberResistance=1e6  SnubberCapacitance=inf  Measurements=None  MoreParameters=on  NoBreakLoop=off
  Constant Power Load : Subsystem
      settings: PortSchema="{\"entries\":[{\"content\":{\"sides\":[{\"content\":{\"connectorIds\":[]},\"type\":\"ConnectorPlacement.EquallySpacedRectSide\",\"uuid\":\"d64f8841-075a-4592-9721-07346c3eedde\"},{\"content\":{\"connectorIds\":[],\"side\":\"RIGHT\"},\"type\":\"ConnectorPlacement.EquallySpacedRectSide\",\"uuid\":\"f70d4421-2220-4657-8c99-8abb3184730b\"},{\"content\":{\"connectorIds\":[\"LConn1\"],\"side\":\"TOP\"},\"type\":\"ConnectorPlacement.EquallySpacedRectSide\",\"uuid\":\"2f586390-110d-4cc5-90f4-9aa5cf771f84\"},{\"content\":{\"connectorIds\":[\"RConn1\"],\"side\":\"BOTTOM\"},\"type\":\"ConnectorPlacement.EquallySpacedRectSide\",\"uuid\":\"57b4e366-61ab-45b5-95e6-2e46cf17a950\"}]},\"type\":\"ConnectorPlacement.EquallySpacedConnector\",\"uuid\":\"1143dd7b-038b-41e2-a355-4aaf746039e3\"}],\"packageUris\":[\"http://schema.mathworks.com/mf0/Connector/R2020b\"],\"version\":\"1.0\"}"
  ESS - SW : Subsystem
      settings: PortSchema="{\"entries\":[{\"content\":{\"sides\":[{\"content\":{\"connectorIds\":[]},\"type\":\"ConnectorPlacement.EquallySpacedRectSide\",\"uuid\":\"a366de01-415d-4fc7-8830-9a15956661b9\"},{\"content\":{\"connectorIds\":[],\"side\":\"RIGHT\"},\"type\":\"ConnectorPlacement.EquallySpacedRectSide\",\"uuid\":\"8598060f-9f02-4b93-be08-39bfe2a310b6\"},{\"content\":{\"connectorIds\":[\"LConn1\"],\"side\":\"TOP\"},\"type\":\"ConnectorPlacement.EquallySpacedRectSide\",\"uuid\":\"f1589895-78fb-4c72-b1f6-5b4e7ce7130b\"},{\"content\":{\"connectorIds\":[\"RConn1\"],\"side\":\"BOTTOM\"},\"type\":\"ConnectorPlacement.EquallySpacedRectSide\",\"uuid\":\"0a878aa3-6d51-479d-a764-f7fa1ccbaa9c\"}]},\"type\":\"ConnectorPlacement.EquallySpacedConnector\",\"uuid\":\"4d15ead3-9d78-44e1-8395-50a3f1c02350\"}],\"packageUris\":[\"http://schema.mathworks.com/mf0/Connector/R2020b\"],\"version\":\"1.0\"}"
  Inverter Control : Subsystem
  PV - SW : Subsystem
      settings: PortSchema="{\"entries\":[{\"content\":{\"sides\":[{\"content\":{\"connectorIds\":[]},\"type\":\"ConnectorPlacement.EquallySpacedRectSide\",\"uuid\":\"a366de01-415d-4fc7-8830-9a15956661b9\"},{\"content\":{\"connectorIds\":[],\"side\":\"RIGHT\"},\"type\":\"ConnectorPlacement.EquallySpacedRectSide\",\"uuid\":\"8598060f-9f02-4b93-be08-39bfe2a310b6\"},{\"content\":{\"connectorIds\":[\"LConn1\"],\"side\":\"TOP\"},\"type\":\"ConnectorPlacement.EquallySpacedRectSide\",\"uuid\":\"f1589895-78fb-4c72-b1f6-5b4e7ce7130b\"},{\"content\":{\"connectorIds\":[\"RConn1\"],\"side\":\"BOTTOM\"},\"type\":\"ConnectorPlacement.EquallySpacedRectSide\",\"uuid\":\"0a878aa3-6d51-479d-a764-f7fa1ccbaa9c\"}]},\"type\":\"ConnectorPlacement.EquallySpacedConnector\",\"uuid\":\"4d15ead3-9d78-44e1-8395-50a3f1c02350\"}],\"packageUris\":[\"http://schema.mathworks.com/mf0/Connector/R2020b\"],\"version\":\"1.0\"}"
  RL1 : spsThreePhaseSeriesRLCBranchLib/Three-Phase Series RLC Branch  LConnTagsString=A|B|C  RConnTagsString=A|B|C  BranchType=RL  Resistance=Rf*V2^2/(Sbase)  Inductance=Lf*V2^2/(Sbase)/(w0)  Capacitance=inf  Measurements=None
  SC - SW : Subsystem
      settings: PortSchema="{\"entries\":[{\"content\":{\"sides\":[{\"content\":{\"connectorIds\":[]},\"type\":\"ConnectorPlacement.EquallySpacedRectSide\",\"uuid\":\"a366de01-415d-4fc7-8830-9a15956661b9\"},{\"content\":{\"connectorIds\":[],\"side\":\"RIGHT\"},\"type\":\"ConnectorPlacement.EquallySpacedRectSide\",\"uuid\":\"8598060f-9f02-4b93-be08-39bfe2a310b6\"},{\"content\":{\"connectorIds\":[\"LConn1\"],\"side\":\"TOP\"},\"type\":\"ConnectorPlacement.EquallySpacedRectSide\",\"uuid\":\"f1589895-78fb-4c72-b1f6-5b4e7ce7130b\"},{\"content\":{\"connectorIds\":[\"RConn1\"],\"side\":\"BOTTOM\"},\"type\":\"ConnectorPlacement.EquallySpacedRectSide\",\"uuid\":\"0a878aa3-6d51-479d-a764-f7fa1ccbaa9c\"}]},\"type\":\"ConnectorPlacement.EquallySpacedConnector\",\"uuid\":\"4d15ead3-9d78-44e1-8395-50a3f1c02350\"}],\"packageUris\":[\"http://schema.mathworks.com/mf0/Connector/R2020b\"],\"version\":\"1.0\"}"
  Series RLC Branch1 : spsSeriesRLCBranchLib/Series RLC Branch  LConnTagsString=__new0  RConnTagsString=__new0  BranchType=C  Resistance=0.1  Inductance=3e-3  SetiL0=off  InitialCurrent=0  Capacitance=C  Setx0=on  InitialVoltage=Vdc_nom  Measurements=None
  Three-Phase Parallel RLC Branch1 : spsThreePhaseParallelRLCBranchLib/Three-Phase Parallel RLC Branch  LConnTagsString=A|B|C  RConnTagsString=A|B|C  BranchType=C  Resistance=1/Gf*Vnom^2/(Pnom)  Inductance=1e-3  Capacitance=Cf*(Sbase)/V2^2/(w0)  Measurements=None
  Universal Bridge : spsUniversalBridgeLib/Universal Bridge  Arms=3  SnubberResistance=1e5  SnubberCapacitance=inf  Device=IGBT / Diodes  Ron=1e-4  Lon=0  ForwardVoltages="[  0  0  ]"  ForwardVoltage=0  GTOparameters=[ 10e-6 , 20e-6 ]  IGBTparameters=[ 1e-6 , 2e-6 ]  Measurements=None  Measurements_2=None  converterType=Rectifier
  "V -> pu" : Gain  Gain=1/Vdc_nom
  Voltage Measurement : spsVoltageMeasurementLib/Voltage Measurement  PhasorSimulation=off  OutputType=Complex  PSBequivalent=0
  a : PMIOPort  Side=Right
  b : PMIOPort  Port=2  Side=Right
  c : PMIOPort  Port=3  Side=Right
  Vdc : Outport
  fac : Outport  Port=2
  Vac : Outport  Port=3
  wires:
  B1/1 -> Inverter Control/1(Igabc)
  [Vdc] -> Inverter Control/4(Vdc), "V -> pu"/1
  "V -> pu"/1 -> Vdc/1
  B2/2 -> Inverter Control/3(Iabc)
  B2/1 -> Inverter Control/2(Vabc)
  Inverter Control/3(mabc) -> Universal Bridge/1
  Inverter Control/1(Vac) -> Vac/1
  Inverter Control/2(fac) -> fac/1
  Voltage Measurement/1 -> [Vdc]
  connections:
  RL1/RConn3 -- Universal Bridge/LConn3
  Universal Bridge/LConn2 -- RL1/RConn2
  RL1/RConn1 -- Universal Bridge/LConn1
  c/RConn1 -- B1/RConn3
  B1/RConn2 -- b/RConn1
  a/RConn1 -- B1/RConn1
  Three-Phase Parallel RLC Branch1/LConn1 -- B2/RConn3 -- B1/LConn3
  Three-Phase Parallel RLC Branch1/LConn3 -- B2/RConn1 -- B1/LConn1
  Three-Phase Parallel RLC Branch1/RConn1 -- Three-Phase Parallel RLC Branch1/RConn3 -- Three-Phase Parallel RLC Branch1/RConn2
  SC - SW/LConn1 -- Breaker2/RConn1
  ESS - SW/LConn1 -- Breaker1/RConn1
  PV - SW/LConn1 -- Breaker/RConn1
  Series RLC Branch1/LConn1 -- Universal Bridge/RConn1 -- Breaker/LConn1 -- Breaker1/LConn1 -- Breaker3/LConn1 -- Breaker2/LConn1 -- Voltage Measurement/LConn1
  B1/LConn2 -- B2/RConn2 -- Three-Phase Parallel RLC Branch1/LConn2
  B2/LConn3 -- RL1/LConn3
  B2/LConn2 -- RL1/LConn2
  B2/LConn1 -- RL1/LConn1
  Universal Bridge/RConn2 -- Voltage Measurement/LConn2 -- Constant Power Load/RConn1 -- SC - SW/RConn1 -- ESS - SW/RConn1 -- PV - SW/RConn1 -- Series RLC Branch1/RConn1
  Constant Power Load/LConn1 -- Breaker3/RConn1

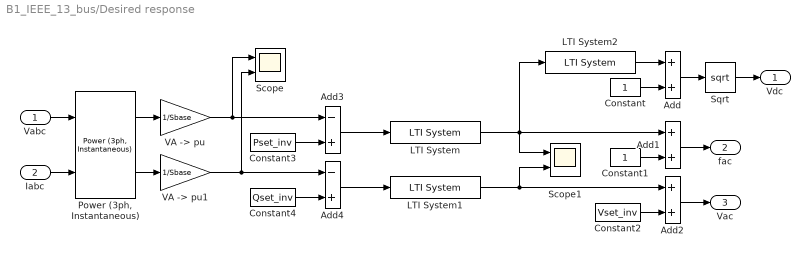
== system B1_IEEE_13_bus/Desired response ==
  Vabc : Inport
  Iabc : Inport  Port=2
  Add : Sum
  Add1 : Sum
  Add2 : Sum
  Add3 : Sum  Inputs=-+
  Add4 : Sum  Inputs=-+
  Constant : Constant
  Constant1 : Constant
  Constant2 : Constant  Value=Vset_inv
  Constant3 : Constant  Value=Pset_inv
  Constant4 : Constant  Value=Qset_inv
  LTI System : cstblocks/LTI System  sys=T_des_fp  IC=[]
  LTI System1 : cstblocks/LTI System  sys=T_des_vq  IC=[]
  LTI System2 : cstblocks/LTI System  sys=T_des_vdcf  IC=[]
  "Power (3ph, Instantaneous)" : spsPower3phInstantaneousLib/Power (3ph, Instantaneous)
  Scope : Scope  NumInputPorts=2
  Scope1 : Scope  NumInputPorts=2
  Sqrt : Sqrt
  "VA -> pu" : Gain  Gain=1/Sbase
  "VA -> pu1" : Gain  Gain=1/Sbase
  Vdc : Outport
  fac : Outport  Port=2
  Vac : Outport  Port=3
  wires:
  Vabc/1 -> "Power (3ph, Instantaneous)"/1
  Iabc/1 -> "Power (3ph, Instantaneous)"/2
  Add3/1 -> LTI System/1
  "Power (3ph, Instantaneous)"/2 -> "VA -> pu1"/1
  LTI System/1 -> Scope1/1, Add1/1, LTI System2/1
  LTI System1/1 -> Scope1/2, Add2/1
  Add/1 -> Sqrt/1
  Constant/1 -> Add/2
  Constant1/1 -> Add1/2
  Add1/1 -> fac/1
  Constant2/1 -> Add2/2
  Add2/1 -> Vac/1
  "Power (3ph, Instantaneous)"/1 -> "VA -> pu"/1
  Add4/1 -> LTI System1/1
  Constant3/1 -> Add3/2
  Constant4/1 -> Add4/2
  "VA -> pu"/1 -> Scope/1, Add3/1
  "VA -> pu1"/1 -> Scope/2, Add4/1
  LTI System2/1 -> Add/1
  Sqrt/1 -> Vdc/1

== system B1_IEEE_13_bus/Double click here for more info ==

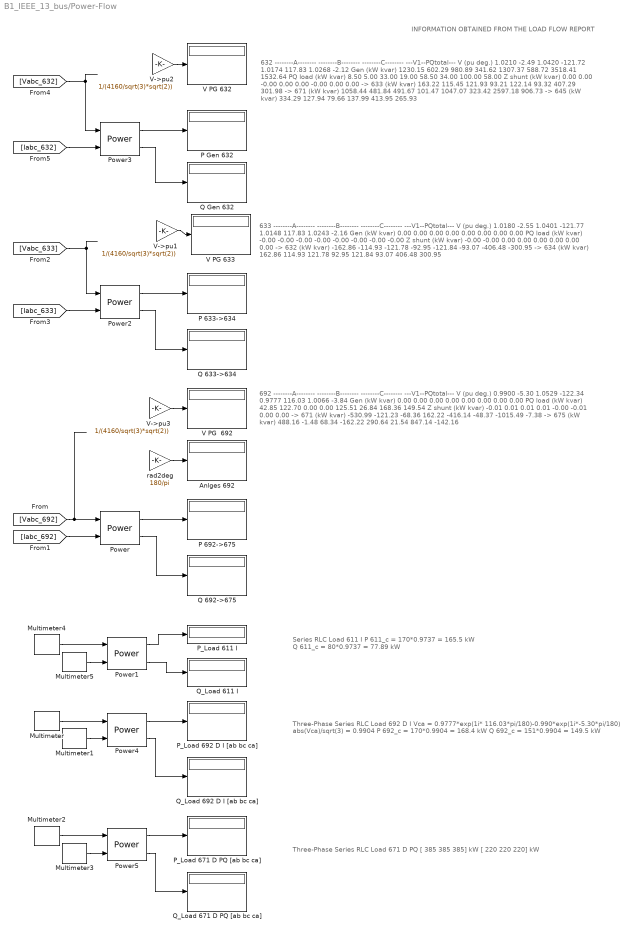
== system B1_IEEE_13_bus/Power-Flow ==
  note: 692 --------A-------- --------B-------- --------C-------- ---V1--PQtotal---
      | V (pu deg.) 0.9900 -5.30 1.0529 -122.34 0.9777 116.03 1.0066 -3.84
      | Gen (kW kvar) 0.00 0.00 0.00 0.00 0.00 0.00 0.00 0.00
      | PQ load (kW kvar) 42.85 122.70 0.00 0.00 125.51 26.84 168.36 149.54
      | Z shunt (kW kvar) -0.01 0.01 0.01 0.01 -0.00 -0.01 0.00 0.00
      |
      | -> 671 (kW kvar) -530.99 -121.23 -68.36 162.22 -416.14 -48.37 -1015.49 -7.38
      | -> 675 (kW kvar) 488.16 -1.48 68.34 -162.22 290.64 21.54 847.14 -142.16
  note: 633 --------A-------- --------B-------- --------C-------- ---V1--PQtotal---
      | V (pu deg.) 1.0180 -2.55 1.0401 -121.77 1.0148 117.83 1.0243 -2.16
      | Gen (kW kvar) 0.00 0.00 0.00 0.00 0.00 0.00 0.00 0.00
      | PQ load (kW kvar) -0.00 -0.00 -0.00 -0.00 -0.00 -0.00 -0.00 -0.00
      | Z shunt (kW kvar) -0.00 -0.00 0.00 0.00 0.00 0.00 0.00 0.00
      |
      | -> 632 (kW kvar) -162.86 -114.93 -121.78 -92.95 -121.84 -93.07 -406.48 -300.95
      | -> 634 (kW kvar) 162.86 114.93 121.78 92.95 121.84 93.07 406.48 300.95
  note: 632 --------A-------- --------B-------- --------C-------- ---V1--PQtotal---
      | V (pu deg.) 1.0210 -2.49 1.0420 -121.72 1.0174 117.83 1.0268 -2.12
      | Gen (kW kvar) 1230.15 602.29 980.89 341.62 1307.37 588.72 3518.41 1532.64
      | PQ load (kW kvar) 8.50 5.00 33.00 19.00 58.50 34.00 100.00 58.00
      | Z shunt (kW kvar) 0.00 0.00 -0.00 0.00 0.00 -0.00 0.00 0.00
      |
      | -> 633 (kW kvar) 163.22 115.45 121.93 93.21 122.14 93.32 407.29 301.98
      | -> 671 (kW kvar) 1058.44 481.84 491.67 101.47 1047.07 323.42 2597.18 906.73
      | -> 645 (kW kvar) 334.29 127.94 79.66 137.99 413.95 265.93
  note: Three-Phase Series RLC Load 671 D PQ
      | [ 385 385 385] kW
      | [ 220 220 220] kW
  note: Three-Phase Series RLC Load 692 D I
      | Vca = 0.9777*exp(1i* 116.03*pi/180)-0.990*exp(1i*-5.30*pi/180)
      | abs(Vca)/sqrt(3) = 0.9904
      | P 692_c = 170*0.9904 = 168.4 kW
      | Q 692_c = 151*0.9904 = 149.5 kW
  note: Series RLC Load 611 I
      | P 611_c = 170*0.9737 = 165.5 kW
      | Q 611_c = 80*0.9737 = 77.89 kW
  note: INFORMATION OBTAINED FROM THE LOAD FLOW REPORT
  Anlges 692 : Display
  Multimeter : spsMultimeterLib/Multimeter  L=26  sel=[8 9 10]  yselected={}  Gain=[1 1 1]  OutputType=Complex  PlotAtSimulationStop=off  PhasorSimulation=off
  Multimeter1 : spsMultimeterLib/Multimeter  L=26  sel=[21 22 23]  yselected={}  Gain=[1 1 1]  OutputType=Complex  PlotAtSimulationStop=off  PhasorSimulation=off
  Multimeter2 : spsMultimeterLib/Multimeter  L=26  sel=[2 3 4]  yselected={}  Gain=[1 1 1]  OutputType=Complex  PlotAtSimulationStop=off  PhasorSimulation=off
  Multimeter3 : spsMultimeterLib/Multimeter  L=26  sel=[15 16 17]  yselected={}  Gain=[1 1 1]  OutputType=Complex  PlotAtSimulationStop=off  PhasorSimulation=off
  Multimeter4 : spsMultimeterLib/Multimeter  L=26  sel=1  yselected={}  Gain=1  OutputType=Complex  PlotAtSimulationStop=off  PhasorSimulation=off
  Multimeter5 : spsMultimeterLib/Multimeter  L=26  sel=14  yselected={}  Gain=1  OutputType=Complex  PlotAtSimulationStop=off  PhasorSimulation=off
  P 633->634 : Display
  P 692->675 : Display
  P Gen 632 : Display
  P_Load 611 I : Display
  P_Load 671 D PQ [ab bc ca] : Display
  P_Load 692 D I [ab bc ca] : Display
  Power{,1..5} (6 alike) : spsPowerLib/Power  Freq=60  Vinit=[1, 0]  Iinit=[1, 0]  Ts=0
  Q 633->634 : Display
  Q 692->675 : Display
  Q Gen 632 : Display
  Q_Load 611 I : Display
  Q_Load 671 D PQ [ab bc ca] : Display
  Q_Load 692 D I [ab bc ca] : Display
  V PG  692 : Display
  V PG 632 : Display
  V PG 633 : Display
  V->pu1 : Gain  Gain=1/(4160/sqrt(3)*sqrt(2))
  V->pu2 : Gain  Gain=1/(4160/sqrt(3)*sqrt(2))
  V->pu3 : Gain  Gain=1/(4160/sqrt(3)*sqrt(2))
  rad2deg : Gain  Gain=180/pi
  wires:
  V->pu3/1 -> V PG  692/1
  Power1/2 -> Q_Load 611 I/1
  Power1/1 -> P_Load 611 I/1
  Multimeter5/1 -> Power1/2
  Multimeter4/1 -> Power1/1
  rad2deg/1 -> Anlges 692/1
  ? -> rad2deg/1
  [Vabc_692] -> Power/1
  ? -> V->pu3/1
  Power5/2 -> Q_Load 671 D PQ [ab bc ca]/1
  Power5/1 -> P_Load 671 D PQ [ab bc ca]/1
  Multimeter3/1 -> Power5/2
  Multimeter2/1 -> Power5/1
  Power4/2 -> Q_Load 692 D I [ab bc ca]/1
  Power4/1 -> P_Load 692 D I [ab bc ca]/1
  Multimeter1/1 -> Power4/2
  Multimeter/1 -> Power4/1
  V->pu2/1 -> V PG 632/1
  [Vabc_632] -> Power3/1
  Power3/2 -> Q Gen 632/1
  Power3/1 -> P Gen 632/1
  [Iabc_632] -> Power3/2
  V->pu1/1 -> V PG 633/1
  [Vabc_633] -> Power2/1
  Power2/2 -> Q 633->634/1
  Power2/1 -> P 633->634/1
  [Iabc_633] -> Power2/2
  Power/2 -> Q 692->675/1
  Power/1 -> P 692->675/1
  [Iabc_692] -> Power/2
  ? -> V->pu2/1
  ? -> V->pu1/1

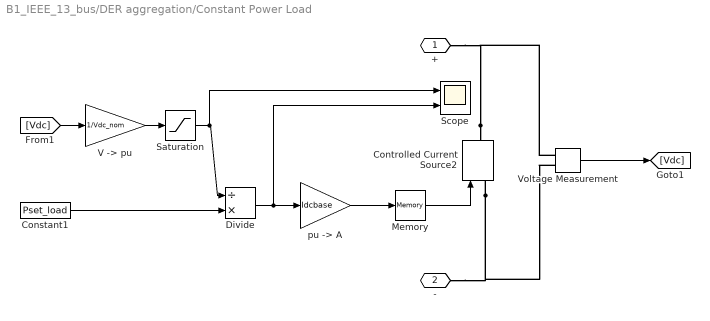
== system B1_IEEE_13_bus/DER aggregation/Constant Power Load ==
  Constant1 : Constant  Value=Pset_load
  Controlled Current Source2 : spsControlledCurrentSourceLib/Controlled Current Source  Initialize=on  Source_Type=DC  Amplitude=0  Phase=0  Frequency=0  Measurements=None
  Divide : Product  Inputs=/*
  Memory : Memory
  Saturation : Saturate  UpperLimit=1.5  LowerLimit=0.5
  Scope : Scope  NumInputPorts=2
  "V -> pu" : Gain  Gain=1/Vdc_nom
  Voltage Measurement : spsVoltageMeasurementLib/Voltage Measurement  PhasorSimulation=off  OutputType=Complex  PSBequivalent=0
  "pu -> A" : Gain  Gain=Idcbase
  + : PMIOPort  Side=Left
  - : PMIOPort  Port=2  Side=Right
  wires:
  "V -> pu"/1 -> Saturation/1
  Saturation/1 -> Scope/1, Divide/1
  Constant1/1 -> Divide/2
  "pu -> A"/1 -> Memory/1
  Divide/1 -> Scope/2, "pu -> A"/1
  [Vdc] -> "V -> pu"/1
  Voltage Measurement/1 -> [Vdc]
  Memory/1 -> Controlled Current Source2/1
  connections:
  Controlled Current Source2/RConn1 -- Voltage Measurement/LConn1 -- +/RConn1
  Controlled Current Source2/LConn1 -- Voltage Measurement/LConn2 -- -/RConn1
